simulink model "TrafficLightSystemWithTestHarness"  (R2020a)
settings: Solver=FixedStepAuto  StartTime=0.0  StopTime=500  FixedStep=0.2  RelTol=1e-3
undefined symbols (not defined in the file): sigbuilder_block
settings Model: EnablePacing=on  PacingRate=22  Creator=Arsal Abbas  LastModifiedBy=Arsal Abbas
settings OptimizationCC: LifeSpan=inf
settings DebuggingCC: ArithmeticOperatorsInVariantConditions=warning
settings SFSimCC: CustomCodeUndefinedFunction=UseInterfaceOnly
settings CodeAppCC: StateflowObjectComments=on

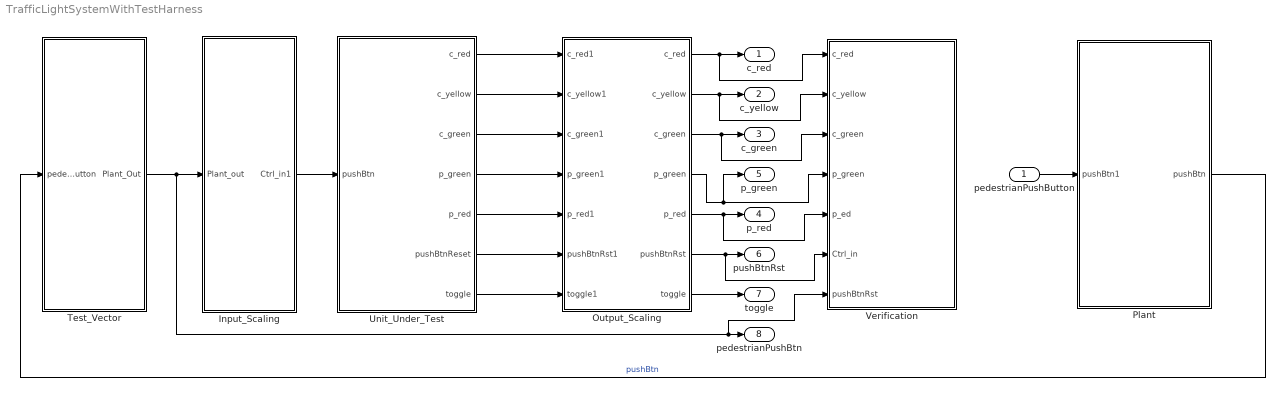
== system TrafficLightSystemWithTestHarness ==
  pedestrianPushButton : Inport
  Input_Scaling : Subsystem
  Output_Scaling : Subsystem
  Plant : Subsystem
  Test_Vector : Subsystem
  Unit_Under_Test : Subsystem
  Verification : Subsystem
  c_red : Outport
  c_yellow : Outport  Port=2
  c_green : Outport  Port=3
  p_red : Outport  Port=4
  p_green : Outport  Port=5
  pushBtnRst : Outport  Port=6
  toggle : Outport  Port=7
  pedestrianPushBtn : Outport  Port=8
  wires:
  Plant/1(pushBtn) -> Test_Vector/1(pedestrianPushButton)  "pushBtn"
  Input_Scaling/1(Ctrl_in1) -> Unit_Under_Test/1(pushBtn)
  pedestrianPushButton/1 -> Plant/1(pushBtn1)
  Test_Vector/1(Plant_Out) -> Verification/7(pushBtnRst), pedestrianPushBtn/1, Input_Scaling/1(Plant_out)
  Unit_Under_Test/1(c_red) -> Output_Scaling/1(c_red1)
  Unit_Under_Test/2(c_yellow) -> Output_Scaling/2(c_yellow1)
  Unit_Under_Test/3(c_green) -> Output_Scaling/3(c_green1)
  Unit_Under_Test/4(p_green) -> Output_Scaling/4(p_green1)
  Unit_Under_Test/5(p_red) -> Output_Scaling/5(p_red1)
  Unit_Under_Test/6(pushBtnReset) -> Output_Scaling/6(pushBtnRst1)
  Unit_Under_Test/7(toggle) -> Output_Scaling/7(toggle1)
  Output_Scaling/1(c_red) -> Verification/1(c_red), c_red/1
  Output_Scaling/2(c_yellow) -> Verification/2(c_yellow), c_yellow/1
  Output_Scaling/3(c_green) -> Verification/3(c_green), c_green/1
  Output_Scaling/5(p_red) -> Verification/5(p_ed), p_red/1
  Output_Scaling/4(p_green) -> Verification/4(p_green), p_green/1
  Output_Scaling/6(pushBtnRst) -> Verification/6(Ctrl_in), pushBtnRst/1
  Output_Scaling/7(toggle) -> toggle/1

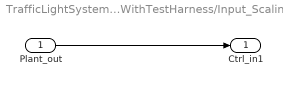
== system TrafficLightSystemWithTestHarness/Input_Scaling ==
  Plant_out : Inport
  Ctrl_in1 : Outport
  wires:
  Plant_out/1 -> Ctrl_in1/1

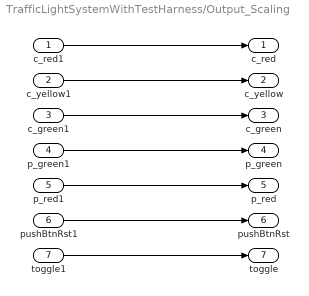
== system TrafficLightSystemWithTestHarness/Output_Scaling ==
  c_red1 : Inport
  c_yellow1 : Inport  Port=2
  c_green1 : Inport  Port=3
  p_green1 : Inport  Port=4
  p_red1 : Inport  Port=5
  pushBtnRst1 : Inport  Port=6
  toggle1 : Inport  Port=7
  c_red : Outport
  c_yellow : Outport  Port=2
  c_green : Outport  Port=3
  p_green : Outport  Port=4
  p_red : Outport  Port=5
  pushBtnRst : Outport  Port=6
  toggle : Outport  Port=7
  wires:
  pushBtnRst1/1 -> pushBtnRst/1
  c_red1/1 -> c_red/1
  c_yellow1/1 -> c_yellow/1
  p_red1/1 -> p_red/1
  c_green1/1 -> c_green/1
  toggle1/1 -> toggle/1
  p_green1/1 -> p_green/1

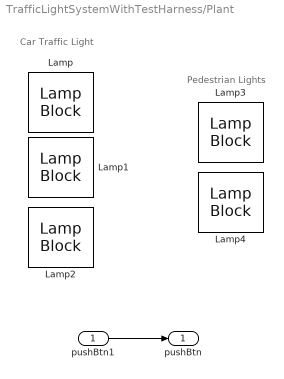
== system TrafficLightSystemWithTestHarness/Plant ==
  note: Car Traffic Light
  note: Pedestrian
      | Lights
  pushBtn1 : Inport
  Lamp{,1..4} (5 alike) : LampBlock
  pushBtn : Outport
  wires:
  pushBtn1/1 -> pushBtn/1

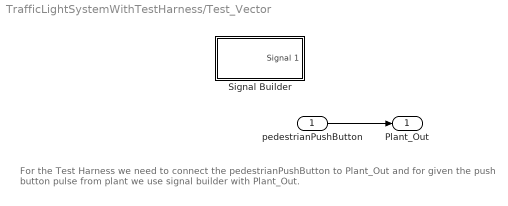
== system TrafficLightSystemWithTestHarness/Test_Vector ==
  note: For the Test Harness we need to connect the pedestrianPushButton to Plant_Out
      | and for given the push button pulse from plant we use signal builder with Plant_Out.
  pedestrianPushButton : Inport
  Signal Builder : Subsystem  Tag=STV Subsys  LoadFcn=sigbuilder_block('load');  StartFcn=sigbuilder_block('start');  StopFcn=sigbuilder_block('stop');  ClipboardFcn=sigbuilder_block('clipboard');  mask(Sigbuilder block){tuvar=[0:10]}
      mask help: Simulink:masks:SigbuilderBlock_MD
      mask init:
      | if ~strcmp(get_param(bdroot(gcbh),'SimulationStatus'),'stopped') tuvar = sigbuilder_block('maskInit'); end
      settings: CopyFcn=sigbuilder_block('copy');  DeleteFcn=sigbuilder_block('delete');  ModelCloseFcn=sigbuilder_block('modelClose');  PreSaveFcn=sigbuilder_block('preSave');  PauseFcn=sigbuilder_block('pause');  ContinueFcn=sigbuilder_block('continue');  NameChangeFcn=sigbuilder_block('namechange');  OpenFcn=sigbuilder_block('open',[437.6 199.2 550.4 400 ]);  CloseFcn=sigbuilder_block('close');
      mask Display: plot(0, 0, 100, 100,[2, 2, 32, 32, 2], [68, 8, 8, 68, 68],[32, 2], [38, 38], [32, 19, 2],[53, 60, 44], [32, 17, 17, 2],[16, 16, 31, 31]);txt = getActiveGroup(gcbh);text(2, 100, txt,'verticalAlignment', 'top');
  Plant_Out : Outport
  wires:
  pedestrianPushButton/1 -> Plant_Out/1

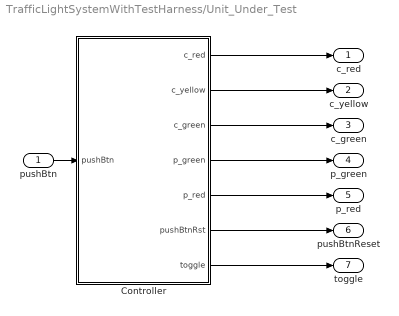
== system TrafficLightSystemWithTestHarness/Unit_Under_Test ==
  pushBtn : Inport
  Controller : Stateflow chart  TreatAsAtomicUnit=on
  c_red : Outport
  c_yellow : Outport  Port=2
  c_green : Outport  Port=3
  p_green : Outport  Port=4
  p_red : Outport  Port=5
  pushBtnReset : Outport  Port=6
  toggle : Outport  Port=7
  wires:
  Controller/3(c_green) -> c_green/1
  Controller/2(c_yellow) -> c_yellow/1
  Controller/1(c_red) -> c_red/1
  pushBtn/1 -> Controller/1(pushBtn)
  Controller/4(p_green) -> p_green/1
  Controller/5(p_red) -> p_red/1
  Controller/6(pushBtnRst) -> pushBtnReset/1
  Controller/7(toggle) -> toggle/1

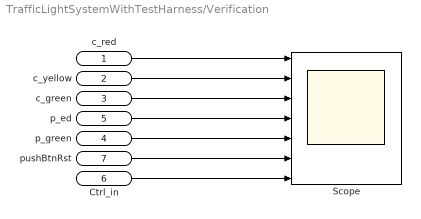
== system TrafficLightSystemWithTestHarness/Verification ==
  c_red : Inport
  c_yellow : Inport  Port=2
  c_green : Inport  Port=3
  p_green : Inport  Port=4
  p_ed : Inport  Port=5
  Ctrl_in : Inport  Port=6
  pushBtnRst : Inport  Port=7
  Scope : Scope  NumInputPorts=7
  wires:
  c_red/1 -> Scope/1
  c_green/1 -> Scope/3
  c_yellow/1 -> Scope/2
  p_ed/1 -> Scope/4
  p_green/1 -> Scope/5
  Ctrl_in/1 -> Scope/7
  pushBtnRst/1 -> Scope/6

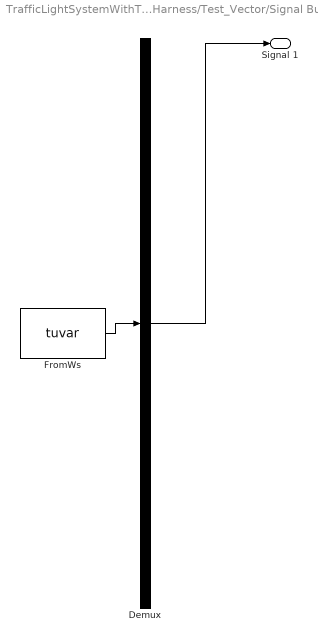
== system TrafficLightSystemWithTestHarness/Test_Vector/Signal Builder ==
  Demux : Demux  Tag=STV Demux  Outputs=1
      settings: DisplayOption=none
  FromWs : FromWorkspace  Tag=STV FromWs  VariableName=tuvar
      SigBuilderData=|
      | common.afterFinalStr = 'Extrapolate'
      | common.sampleTime = 0
      | dataSet.timeRange = [0 10]
      | dataSet.name = 'Group 1'
      | sbobj.Groups.Name = 'Group 1'
      | sbobj.Groups.Signals.Name = 'Signal 1'
      | sbobj.Groups.Signals.XData = [0 4 4 6 6 10]
      | sbobj.Groups.Signals.YData = [0 0 1 1 0 0]
  Signal 1 : Outport  Tag=STV Outport
  wires:
  Demux/1 -> Signal 1/1
  FromWs/1 -> Demux/1

== stateflow chart TrafficLightSystemWithTestHarness/Unit_Under_Test/Controller ==
  state TraffcLight [parallel]
    settings: executionOrder=1
    state P_Green
      entry:
      pushBtnRst=1;
      p_green=1;
      during:
      p_green=1;
      toggle=0;
      exit:
      p_green =0;
      p_red=1;
      toggle=0;
    state Car_RedYellow
      entry:
      p_red=1;
      c_red = 1;
      c_yellow = 1;
      during:
      c_red = 1;
      c_yellow = 1;
      p_green=0;
      exit:
      c_red = 0;
      c_yellow = 0;
      p_green=0;
      p_red=1;
    state Car_Red
      entry:
      c_red = 1;
      during:
      c_red = 1;
      on after (10,sec):
      toggle=0;
      exit:
      c_red = 1;
      state P_Red
        entry:
        pushBtnRst=0;
        p_red=1;
        during:
        p_red=1;
        exit:
        p_red=0;
      (default) -> P_Red
    state Car_Green
      entry:
      c_green = 1;
      during:
      c_green = 1;
      p_green=0;
      p_red=1;
      exit:
      c_green = 0;
      p_green=0;
      p_red=1;
    state Car_Yellow
      entry:
      c_yellow = 1;
      during:
      c_yellow = 1;
      p_green=0;
      p_red=1;
      exit:
      c_yellow = 0;
      p_green=0;
      p_red=1;
    (junction 65) -> P_Green : after(5,sec)[toggle==1 && c_red==1]
    P_Red -> (junction 65)
    P_Green -> (junction 67)
    (junction 67) -> (junction 74) : after(20,sec)/{toggle==0}
    (default) -> Car_Red
    (junction 74) -> Car_RedYellow
    Car_Green -> Car_Yellow : after(30,sec)/{p_red==1}
    Car_Yellow -> Car_Red : after(5,sec)
    Car_Red -> Car_RedYellow : after(30,sec)/{p_red==1 }
    (junction 23) -> Car_Green
    Car_RedYellow -> (junction 21)
    (junction 21) -> (junction 23) : after(5,sec)
  state Toggle [parallel]
    settings: executionOrder=2
    state toggleOn1
      entry:
      toggle=1;
      during:
      toggle=1;
      exit:
      toggle=0
    state toggleOff
      entry:
      toggle=0;
      during:
      toggle=0;
      exit:
      toggle=0;
    (default) -> toggleOff
    toggleOn1 -> toggleOff : [pushBtn==0 && pushBtnRst==1]
    toggleOff -> toggleOn1 : [pushBtn==1 && pushBtnRst==0]
  data: c_red output; c_yellow output; c_green output; pushBtn input; p_green output; p_red output; pushBtnRst output; toggle output
